simulink model "Carla"  (R2019a)
settings: Solver=VariableStepAuto  StartTime=0.0  StopTime=inf  RelTol=1e-3
libraries: visionsinks x2
settings Model: Creator=darks  LastModifiedBy=darks

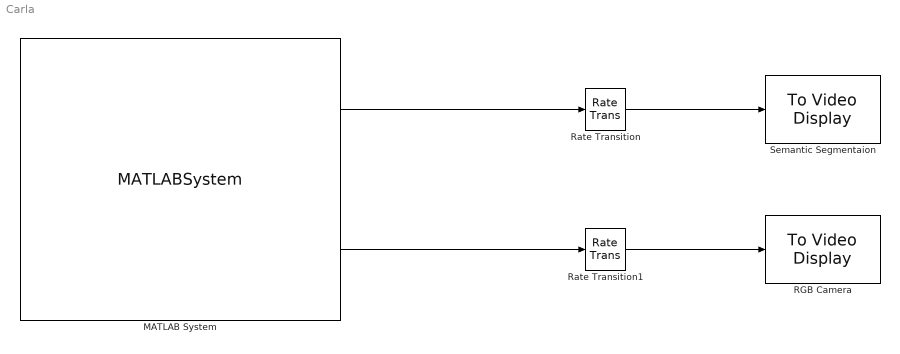
== system Carla ==
  MATLAB System : MATLABSystem  System=CarlaEnvironment  SimulateUsing=Interpreted execution
      mask Type: CarlaEnvironment
      mask Display:
      | disp('CarlaEnvironment');
      | port_label('output',1,'SEMANTIC_SEGMENTATION_RGB');
      | port_label('output',2,'RGB');
  RGB Camera : visionsinks/To Video Display  windowSizeMode=Normal  openAtMdlStart=on  fullScreen=off  videoWindowX=536805376  videoWindowY=536805376  saveWindowSize=off  videoWindowWidth=2147483647  videoWindowHeight=2147483647  inputColorFormat=RGB  inputType=Obsolete  imagePorts=One multidimensional signal  OutputDevice=On-screen video monitor  dataOrg=Column-major  isWindowOpen=off
      settings: SourceProductName=Computer Vision Toolbox
  Rate Transition : RateTransition  OutPortSampleTime=.1
  Rate Transition1 : RateTransition  OutPortSampleTime=.1
  Semantic Segmentaion : visionsinks/To Video Display  windowSizeMode=Normal  openAtMdlStart=on  fullScreen=off  videoWindowX=536805376  videoWindowY=536805376  saveWindowSize=off  videoWindowWidth=2147483647  videoWindowHeight=2147483647  inputColorFormat=RGB  inputType=Obsolete  imagePorts=One multidimensional signal  OutputDevice=On-screen video monitor  dataOrg=Column-major  isWindowOpen=off
      settings: SourceProductName=Computer Vision Toolbox
  wires:
  Rate Transition/1 -> Semantic Segmentaion/1
  MATLAB System/1 -> Rate Transition/1
  MATLAB System/2 -> Rate Transition1/1
  Rate Transition1/1 -> RGB Camera/1
